simulink model "tailsitter_simulation_cascaded"  (R2021a)
settings: Solver=VariableStepAuto  StartTime=0.0  StopTime=tf  RelTol=1e-3
values from neighbouring files (symbols this model uses):
  b = 0.6    [linear_dynamics_hover.m]    (also in nonlinear_dynamics_eq.m; simulink_setup.m; tailsitter.m; tailsitter_sym.m)
  c_bar = 0.142    [linear_dynamics_hover.m]    (also in nonlinear_dynamics_eq.m; simulink_setup.m; tailsitter.m; tailsitter_sym.m)
  CD_f = 0.000762    [linear_dynamics_hover.m]    (also in nonlinear_dynamics_eq.m; simulink_setup.m; tailsitter.m; tailsitter_sym.m)
  CL_0 = 0    [linear_dynamics_hover.m]    (also in nonlinear_dynamics_eq.m; simulink_setup.m; tailsitter.m; tailsitter_sym.m)
  CL_f = 0.036    [linear_dynamics_hover.m]    (also in nonlinear_dynamics_eq.m; simulink_setup.m; tailsitter.m; tailsitter_sym.m)
  Cl_f = 0.0057    [linear_dynamics_hover.m]    (also in nonlinear_dynamics_eq.m; simulink_setup.m; tailsitter.m; tailsitter_sym.m)
  Cm_0 = 0    [linear_dynamics_hover.m]    (also in nonlinear_dynamics_eq.m; simulink_setup.m; tailsitter.m; tailsitter_sym.m)
  Cm_f = -0.0102    [linear_dynamics_hover.m]    (also in nonlinear_dynamics_eq.m; simulink_setup.m; tailsitter.m; tailsitter_sym.m)
  CP = 0.01    [linear_dynamics_hover.m]    (also in nonlinear_dynamics_eq.m; simulink_setup.m; tailsitter.m; tailsitter_sym.m)
  CT = 0.05    [linear_dynamics_hover.m]    (also in nonlinear_dynamics_eq.m; simulink_setup.m; tailsitter.m; tailsitter_sym.m)
  D = 0.12    [linear_dynamics_hover.m]    (also in nonlinear_dynamics_eq.m; simulink_setup.m; tailsitter.m; tailsitter_sym.m)
  dt = 0.005    [simulink_setup.m]    (also in tailsitter_test.m)
  g = 9.81    [linear_dynamics_hover.m]    (also in nonlinear_dynamics_eq.m; simulink_setup.m; tailsitter.m; tailsitter_sym.m)
  J = [Jxx 0 -Jxz; 0 Jyy 0; -Jxz 0 Jzz]    [linear_dynamics_hover.m]    (also in nonlinear_dynamics_eq.m; simulink_setup.m; tailsitter.m; tailsitter_sym.m)
  Kd = 0.01    [simulink_setup.m]
  Kh = -1    [simulink_setup.m]
  Khi = -0.1    [simulink_setup.m]
  Kp = 1    [simulink_setup.m]    (also in tailsitter_test.m = 10)
  Kpi = 10    [simulink_setup.m]    (also in tailsitter_test.m = 100)
  Kq = 1    [simulink_setup.m]    (also in tailsitter_test.m = 10)
  Kqi = 20    [simulink_setup.m]    (also in tailsitter_test.m = 50)
  Kr = 5    [simulink_setup.m]    (also in tailsitter_test.m = 10)
  Kri = 20    [simulink_setup.m]    (also in tailsitter_test.m = 5)
  Kt = -5    [simulink_setup.m]    (also in tailsitter_test.m)
  Kti = -100    [simulink_setup.m]    (also in tailsitter_test.m)
  Ku = -2    [simulink_setup.m]
  Kui = -2    [simulink_setup.m]
  Kv = 5    [simulink_setup.m]
  Kvi = 4    [simulink_setup.m]
  Kw = 1    [simulink_setup.m]
  Kx = 0.2    [simulink_setup.m]
  Ky = 0.2    [simulink_setup.m]
  m = 0.3    [linear_dynamics_hover.m]    (also in nonlinear_dynamics_eq.m; simulink_setup.m; tailsitter.m; tailsitter_sym.m)
  M_flap = [-1 1; -1 -1]    [simulink_setup.m]    (also in tailsitter_test.m)
  M_motor = [1 1; 1 -1]    [simulink_setup.m]    (also in tailsitter_test.m)
  motor_eq = xeq(end)    [simulink_setup.m]
  prop_arm = 0.15    [linear_dynamics_hover.m]    (also in nonlinear_dynamics_eq.m; simulink_setup.m; tailsitter.m; tailsitter_sym.m)
  rho = 1.225    [linear_dynamics_hover.m]    (also in nonlinear_dynamics_eq.m; simulink_setup.m; tailsitter.m; tailsitter_sym.m)
  S_w = S_w/3    (= 0.0276)    [linear_dynamics_hover.m]    (also in nonlinear_dynamics_eq.m; simulink_setup.m = 0.0828; tailsitter.m = 0.0828; tailsitter_sym.m)
  z0 = -2    [simulink_setup.m]
libraries: pid_lib x10, sharedtransform x5, vrlib x3, simulink x2, aerolibutil x2, simulink_extras x1, sharedutil x1
(part 2 of 2)

== system tailsitter_simulation_cascaded/Tailsitter Plant/Aerodynamics/Roll Moment ==
  Input : Inport
  Demux : Demux
  Gain9 : Gain  Gain=S_w/2*b*Cl_f
  Product6 : Product
  Product7 : Product
  Sum7 : Sum  Inputs=|+-
  Out1 : Outport
  wires:
  Sum7/1 -> Gain9/1
  Product7/1 -> Sum7/2
  Product6/1 -> Sum7/1
  Gain9/1 -> Out1/1
  Demux/4 -> Product7/2
  Input/1 -> Demux/1
  Demux/2 -> Product7/1
  Demux/1 -> Product6/1
  Demux/3 -> Product6/2

== system tailsitter_simulation_cascaded/Tailsitter Plant/Aerodynamics/drag ==
  Input : Inport
  Abs : Abs
  Abs1 : Abs
  Demux : Demux
  Gain1 : Gain  Gain=-S_w/2*CD_f
  Gain3 : Gain  Gain=-S_w/2*CD_f
  Product1 : Product
  Product2 : Product
  Sum : Sum  Inputs=|++
  drag : Outport
  wires:
  Demux/3 -> Product2/2
  Abs/1 -> Gain3/1
  Gain3/1 -> Product2/1
  Product2/1 -> Sum/1
  Demux/1 -> Abs/1
  Input/1 -> Demux/1
  Gain1/1 -> Product1/1
  Abs1/1 -> Gain1/1
  Demux/2 -> Abs1/1
  Demux/4 -> Product1/2
  Product1/1 -> Sum/2
  Sum/1 -> drag/1
